simulink model "SCADA_Sawmill"  (R2024b)
settings: Solver=FixedStepAuto  StartTime=0.0  StopTime=Tsim  FixedStep=dT  RelTol=1e-3
values from neighbouring files (symbols this model uses):
  b = t + 2*s    (= 3.6)    [ParametriSegheria.m]    (also in ParametriSegheriaDinamica.m; main_param_CLASSIC.m; main_param_SCADA.m)
  change_cost = 60    [ParametriSegheriaDinamica.m]    (also in main_param_CLASSIC.m = 50; main_param_SCADA.m = 50)
  dT = 0.025    [ParametriSegheriaDinamica.m]    (also in main_param_CLASSIC.m; main_param_SCADA.m)
  h_index = [70, 80, 90, 100]    [ParametriSegheria.m]    (also in ParametriSegheriaDinamica.m = [80, 90, 100]; main_param_CLASSIC.m = [80, 90, 100, 110]; main_param_SCADA.m = [80, 90, 100, 110])
  h_start_1 = 1    [main_param_CLASSIC.m]
  h_start_2 = 2    [main_param_CLASSIC.m]
  h_start_3 = 3    [main_param_CLASSIC.m]
  h_start_4 = 1    [main_param_CLASSIC.m]
  h_start_5 = 2    [main_param_CLASSIC.m]
  h_start_6 = 3    [main_param_CLASSIC.m]
  J1 = 8*1e6    (= 8000000)    [ParametriSegheriaDinamica.m]    (also in main_param_CLASSIC.m; main_param_SCADA.m)
  J2 = 0.9*1e6    (= 900000)    [ParametriSegheriaDinamica.m]    (also in main_param_CLASSIC.m; main_param_SCADA.m)
  kc = [0 35 40 50 55 90]    [ParametriSegheria.m]    (also in ParametriSegheriaDinamica.m = [0, 25, 30, 35, 50, 70]; main_param_CLASSIC.m = [0, 25, 30, 35, 50, 70]; main_param_SCADA.m = [0, 25, 30, 35, 50, 70])
  Kt = 2    [ParametriSegheria.m]    (also in ParametriSegheriaDinamica.m = 10000; main_param_CLASSIC.m = 10000; main_param_SCADA.m = 10000)
  Kt2 = 5    [ParametriSegheria.m]    (also in ParametriSegheriaDinamica.m = 4500; main_param_CLASSIC.m = 4500; main_param_SCADA.m = 4500)
  l_index = [20, 30, 40, 50]    [ParametriSegheria.m]    (also in ParametriSegheriaDinamica.m = [30, 40, 50]; main_param_CLASSIC.m = [30, 40, 50, 60]; main_param_SCADA.m = [30, 40, 50, 60])
  l_start_1 = 1    [main_param_CLASSIC.m]
  l_start_2 = 1    [main_param_CLASSIC.m]
  l_start_3 = 1    [main_param_CLASSIC.m]
  l_start_4 = 1    [main_param_CLASSIC.m]
  l_start_5 = 1    [main_param_CLASSIC.m]
  l_start_6 = 1    [main_param_CLASSIC.m]
  Lt = 4    [ParametriSegheria.m]    (also in ParametriSegheriaDinamica.m; main_param_CLASSIC.m; main_param_SCADA.m)
  Mag_D1 = [0 randi([220 500], 1, 40)]    [ParametriSegheria.m]    (also in ParametriSegheriaDinamica.m = [0 randi([200 500], 1, N_log)]; main_param_CLASSIC.m = [0 randi([200 500], 1, N_log)]; main_param_SCADA.m = [0 randi([200 500], 1, N_log)])
  Mag_D2 = [0 randi([220 500], 1, 40)]    [ParametriSegheria.m]    (also in ParametriSegheriaDinamica.m = [0 randi([200 500], 1, N_log)]; main_param_CLASSIC.m = [0 randi([200 500], 1, N_log)]; main_param_SCADA.m = [0 randi([200 500], 1, N_log)])
  Mag_D3 = [0 randi([220 500], 1, 40)]    [ParametriSegheria.m]    (also in ParametriSegheriaDinamica.m = [0 randi([200 500], 1, N_log)]; main_param_CLASSIC.m = [0 randi([200 500], 1, N_log)]; main_param_SCADA.m = [0 randi([200 500], 1, N_log)])
  Mag_legno1 = [0 randi([1 5], 1, 40)]    [ParametriSegheria.m]    (also in ParametriSegheriaDinamica.m = [0 randi([1 5], 1, N_log)]; main_param_CLASSIC.m = [0 randi([1 5], 1, N_log)]; main_param_SCADA.m = [0 randi([1 5], 1, N_log)])
  Mag_legno2 = [0 randi([1 5], 1, 40)]    [ParametriSegheria.m]    (also in ParametriSegheriaDinamica.m = [0 randi([1 5], 1, N_log)]; main_param_CLASSIC.m = [0 randi([1 5], 1, N_log)]; main_param_SCADA.m = [0 randi([1 5], 1, N_log)])
  Mag_legno3 = [0 randi([1 5], 1, 40)]    [ParametriSegheria.m]    (also in ParametriSegheriaDinamica.m = [0 randi([1 5], 1, N_log)]; main_param_CLASSIC.m = [0 randi([1 5], 1, N_log)]; main_param_SCADA.m = [0 randi([1 5], 1, N_log)])
  n_linee = 3    [ParametriSegheriaDinamica.m]    (also in main_param_CLASSIC.m; main_param_SCADA.m)
  omega_ref1 = 50    [ParametriSegheriaDinamica.m]    (also in main_param_CLASSIC.m; main_param_SCADA.m)
  omega_ref2 = 3000*(2*pi/60)    (= 314.159265359)    [ParametriSegheriaDinamica.m]    (also in main_param_CLASSIC.m; main_param_SCADA.m)
  Rc = 200    [ParametriSegheria.m]    (also in ParametriSegheriaDinamica.m; main_param_CLASSIC.m; main_param_SCADA.m)
  rho = [0, 450, 520, 590, 710, 780]*1e-9    [ParametriSegheriaDinamica.m]    (also in main_param_CLASSIC.m; main_param_SCADA.m)
  Rs = 800    [ParametriSegheria.m]    (also in ParametriSegheriaDinamica.m; main_param_CLASSIC.m; main_param_SCADA.m)
  sigma_D = 10    [ParametriSegheriaDinamica.m]    (also in main_param_CLASSIC.m = 5; main_param_SCADA.m = 5)
  sigma_larg = 10    [ParametriSegheriaDinamica.m]    (also in main_param_CLASSIC.m = 5; main_param_SCADA.m = 5)
  SR = Rs/Rm    (= 5.33333333333)    [ParametriSegheria.m]    (also in ParametriSegheriaDinamica.m; main_param_CLASSIC.m; main_param_SCADA.m)
  SR2 = Rc/Rm2    (= 4)    [ParametriSegheria.m]    (also in ParametriSegheriaDinamica.m; main_param_CLASSIC.m; main_param_SCADA.m)
  target_matrice = randi([20, 120], length(h_index), length(l_index))    [ParametriSegheria.m]    (also in ParametriSegheriaDinamica.m = randi([20, 100], length(h_index), length(l_index)); main_param_CLASSIC.m = randi([20, 100], length(h_index), length(l_index)); main_param_SCADA.m = randi([20, 100], length(h_index), length(l_index)))
  thr_lavoro = 600000    [ParametriSegheriaDinamica.m]    (also in main_param_CLASSIC.m; main_param_SCADA.m)
  V_mean1 = 0.75    [ParametriSegheriaDinamica.m]    (also in main_param_CLASSIC.m; main_param_SCADA.m)
  V_mean23 = 1    [ParametriSegheriaDinamica.m]    (also in main_param_CLASSIC.m; main_param_SCADA.m)
libraries: simulink x24, slpidlib x18
(part 5 of 5)

== matlab function SCADA_Sawmill/Controllo Magazzino/NON INTELLIGENTE ==
  data: h_next output; Magazzino output; stop output; l_next output; h_idx input; target_matrice parameter; n_assi input; l_idx input; change_cost parameter; flag output
function [h_next, Magazzino, stop, l_next, flag] = fcn(h_idx, target_matrice, n_assi, l_idx, change_cost)

[n_rows, n_cols] = size(target_matrice);

h_next = zeros(1,length(h_idx));
l_next = zeros(1,length(l_idx));

persistent MagazzinoReale




if isempty(MagazzinoReale)
    MagazzinoReale = zeros(n_rows, n_cols);
end

for i = 1:length(n_assi)
    % Output iniziali
    h_next(i) = h_idx(i);
    l_next(i) = l_idx(i);

    MagazzinoReale(h_idx(i), l_idx(i)) = MagazzinoReale(h_idx(i), l_idx(i)) + n_assi(i);
end




% AVVISO QUANDO STO PER FINIRE QUELLA SEZIONE
thr = 5;
diff = zeros(1, length(n_assi));
flag = zeros(1, length(n_assi));

for i = 1:length(n_assi)
    diff(i) = target_matrice(h_idx(i), l_idx(i)) - MagazzinoReale(h_idx(i), l_idx(i));
    if diff(i) <= thr
        flag(i) = 1;
    else 
        flag(i) = 0;
    end
end
    


for i = 1:length(n_assi)
    if MagazzinoReale(h_idx(i), l_idx(i)) >= target_matrice(h_idx(i), l_idx(i)) + 2
        
        h_next(i) = h_idx(i);
        if l_idx(i) <= 4
            if l_idx(i) == 4
                l_next(i) = l_idx(i);
            else
                l_next(i) = l_idx(i) + 1;
            end
        end
        
      

        % best_cost = inf;
        % best_h = h_idx(i);
        % best_l = l_idx(i);
        % 
        % 
        % for h = 1:n_rows
        %     for l = 1:n_cols
        % 
        %         if deficit(h,l) > 0
        % 
        %             % Penalità cambio lama
        %             % Per macchina 2, 4, 6 cambio h, per macchina 1, 3, 5
        %             % cambio l
        %             if mod(i, 2) == 0
        %                 cambio = (h ~= h_idx(i));
        %             else
        %                 cambio = (l ~= l_idx(i));
        %             end
        % 
        %             % Funzione costo
        %             cost = -deficit(h,l) + change_cost*cambio;
        % 
        %             if cost < best_cost
        %                 best_cost = cost;
        %                 best_h = h;
        %                 best_l = l;
        %             end
        %         end
        % 
        %     end
        % end
        % 
        % if best_cost < inf
        %     h_next(i) = best_h;
        %     l_next(i) = best_l;
        % end

    end
end

if MagazzinoReale >= target_matrice
    stop = 1;
else
    stop = 0;
end

Magazzino = MagazzinoReale;
